simulink model "Mehra_fixed"  (R2026a)
settings: Solver=ode15s  StopTime=7  MaxStep=0.005  RelTol=1e-6  AbsTol=1e-8
values from neighbouring files (symbols this model uses):
  f = @(u,B) [ A - (B+1)*u(1) + u(1)^2*u(2) ;  B*u(1) - u(1)^2*u(2) ]    [auto_matlab.m]
  qco = 1    [draw_figure7.m]
  R = 15    [draw_figure7.m]    (also in draw_figure7_chirp.m; x15_pio_figures.m; x15_pio_figures_updated.m)
undefined symbols (not defined in the file or in its folder): Kp, thau
settings Model: Creator=t0900  LastModifiedBy=t0900

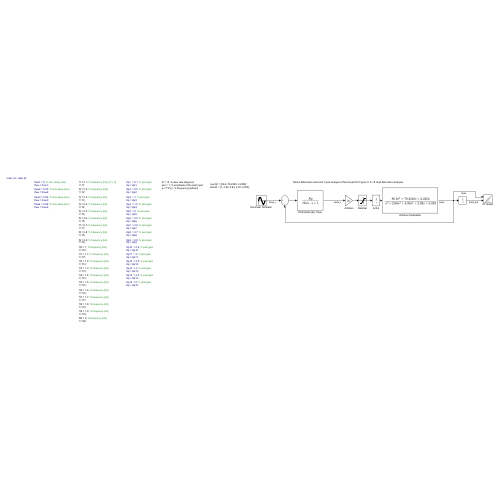
[thumbnail: Simulink's stored preview of the top-level diagram]
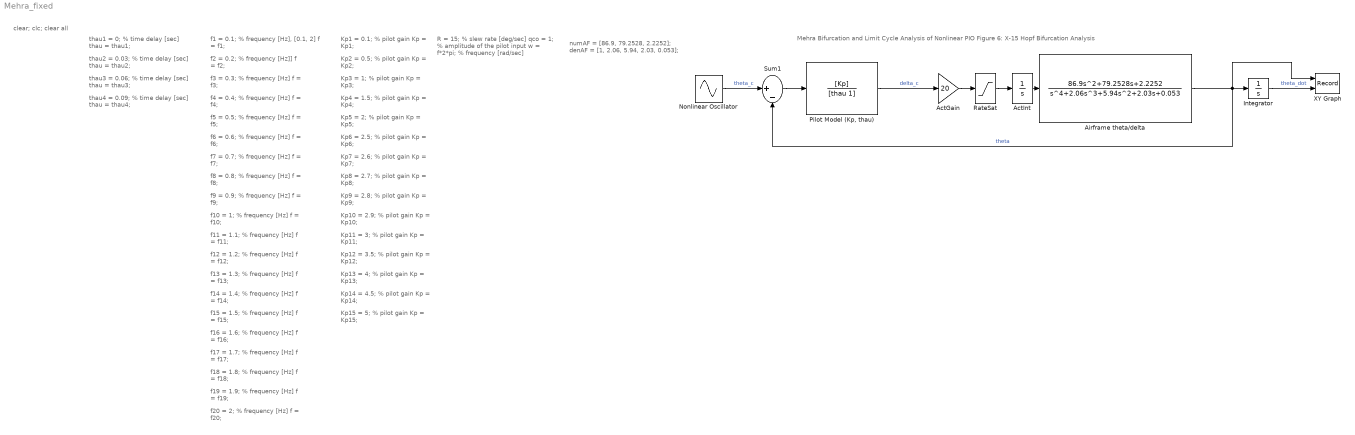
== system Mehra_fixed ==
  note: Kp1  = 0.1; % pilot gain
      | Kp = Kp1;
  note: numAF = [86.9, 79.2528, 2.2252];
      | denAF = [1, 2.06, 5.94, 2.03, 0.053];
  note: R = 15; % slew rate [deg/sec]
      | qco = 1; % amplitude of the pilot input
      | w = f*2*pi; % frequency [rad/sec]
  note: f1 = 0.1; % frequency [Hz], [0.1, 2]
      | f = f1;
  note: thau4 = 0.09; % time delay [sec]
      | thau = thau4;
  note: thau3 = 0.06; % time delay [sec]
      | thau = thau3;
  note: thau2 = 0.03; % time delay [sec]
      | thau = thau2;
  note: thau1 = 0; % time delay [sec]
      | thau = thau1;
  note: Mehra Bifurcation and Limit Cycle Analysis of Nonlinear PIO Figure 6: X-15 Hopf Bifurcation Analysis
  note: clear; clc; clear all
  note: f2 = 0.2; % frequency [Hz]]
      | f = f2;
  note: f3 = 0.3; % frequency [Hz]
      | f = f3;
  note: f4 = 0.4; % frequency [Hz]
      | f = f4;
  note: f5 = 0.5; % frequency [Hz]
      | f = f5;
  note: f6 = 0.6; % frequency [Hz]
      | f = f6;
  note: f7 = 0.7; % frequency [Hz]
      | f = f7;
  note: f8 = 0.8; % frequency [Hz]
      | f = f8;
  note: f9 = 0.9; % frequency [Hz]
      | f = f9;
  note: f10 = 1; % frequency [Hz]
      | f = f10;
  note: f11 = 1.1; % frequency [Hz]
      | f = f11;
  note: f12 = 1.2; % frequency [Hz]
      | f = f12;
  note: f13 = 1.3; % frequency [Hz]
      | f = f13;
  note: f14 = 1.4; % frequency [Hz]
      | f = f14;
  note: f15 = 1.5; % frequency [Hz]
      | f = f15;
  note: f16 = 1.6; % frequency [Hz]
      | f = f16;
  note: f17 = 1.7; % frequency [Hz]
      | f = f17;
  note: f18 = 1.8; % frequency [Hz]
      | f = f18;
  note: f19 = 1.9; % frequency [Hz]
      | f = f19;
  note: f20 = 2; % frequency [Hz]
      | f = f20;
  note: Kp2  = 0.5; % pilot gain
      | Kp = Kp2;
  note: Kp3  = 1; % pilot gain
      | Kp = Kp3;
  note: Kp4  = 1.5; % pilot gain
      | Kp = Kp4;
  note: Kp5  = 2; % pilot gain
      | Kp = Kp5;
  note: Kp6  = 2.5; % pilot gain
      | Kp = Kp6;
  note: Kp7  = 2.6; % pilot gain
      | Kp = Kp7;
  note: Kp8  = 2.7; % pilot gain
      | Kp = Kp8;
  note: Kp9  = 2.8; % pilot gain
      | Kp = Kp9;
  note: Kp10  = 2.9; % pilot gain
      | Kp = Kp10;
  note: Kp11  = 3; % pilot gain
      | Kp = Kp11;
  note: Kp12  = 3.5; % pilot gain
      | Kp = Kp12;
  note: Kp13  = 4; % pilot gain
      | Kp = Kp13;
  note: Kp14  = 4.5; % pilot gain
      | Kp = Kp14;
  note: Kp15  = 5; % pilot gain
      | Kp = Kp15;
  ActGain : Gain  Gain=20
  ActInt : Integrator
  Airframe theta/delta : TransferFcn  Numerator=[86.9, 79.2528, 2.2252]  Denominator=[1, 2.06, 5.94, 2.03, 0.053]
  Integrator : Integrator
  Nonlinear Oscillator : Sin  Amplitude=qco  Frequency=f*2*pi  SampleTime=0
  "Pilot Model (Kp, thau)" : TransferFcn  Numerator=[Kp]  Denominator=[thau 1]
  RateSat : Saturate  UpperLimit=R  LowerLimit=-R
  Sum1 : Sum  Inputs=|+-
  XY Graph : Record  NumPorts=2.0  FileSettingsInternal="{\"entries\":[{\"content\":{\"excelSettings\":{\"content\":{},\"type\":\"Streamout.ExcelSettings\"},\"parquetSettings\":{\"content\":{},\"type\":\"Streamout.ParquetSettings\"}},\"type\":\"Streamout.FileSettingStorage\",\"uuid\":\"\"}],\"packageUris\":[\"http:\\/\\/schema.mathworks.com\\/mf0\\/streamout_blocks\\/R2020a\"],\"version\":\"1.0\"}"  FrameSettings=[0, 0]  Layout=[1 1]  SignalsInternal="{\"entries\":[{\"content\":{\"signals\":[{\"content\":{\"blockPath\":[],\"dimensions\":[1],\"domain\":\"\",\"lineColor\":\"#a2142f\",\"plots\":[ 1 ],\"port\":1,\"signalID\":1,\"signalName\":\"theta\"},\"type\":\"RecordBlkView.Signal\",\"uuid\":\"\"},{\"content\":{\"blockPath\":[],\"dimensions\":[1],\"domain\":\"\",\"lineColor\":\"#139fff\",\"plots\":[ 1 ],\"port\":2,\"signalID\":2,\"signalName\":\"theta_dot\"},\"type\":\"RecordBlkView.Signal\",\"uuid\":\"\"}]},\"type\":\"RecordBlkView.InputSignals\",\"uuid\":\"\"}],\"packageUris\":[\"http:\\/\\/schema.mathworks.com\\/mf0\\/streamout_blocks\\/R2020a\"],\"version\":\"1.0\"}"  VisualizationBindings="{\"xyplotplugin\":{\"info\":[{\"series\":[{\"bindingParametersList\":[{\"parameter\":\"X-Axis\",\"signalID\":1,\"signalName\":\"theta\"},{\"parameter\":\"Y-Axis\",\"signalID\":2,\"signalName\":\"theta_dot\"}],\"seriesID\":0}],\"subplotID\":1}]}}"  CompatibilityTag=XY
  wires:
  Sum1/1 -> "Pilot Model (Kp, thau)"/1
  "Pilot Model (Kp, thau)"/1 -> ActGain/1  "delta_c"
  Nonlinear Oscillator/1 -> Sum1/1  "theta_c"
  Airframe theta/delta/1 -> XY Graph/1, Sum1/2, Integrator/1  "theta"
  Integrator/1 -> XY Graph/2  "theta_dot"
  ActGain/1 -> RateSat/1
  RateSat/1 -> ActInt/1
  ActInt/1 -> Airframe theta/delta/1
